simulink model "inventerthreephase"  (Simulink 7.3)
settings: Solver=ode45  StartTime=0.0  StopTime=0.2  RelTol=1e-3
libraries: powerlib x16
settings Model: Creator=Administrator  LastModifiedBy=Administrator

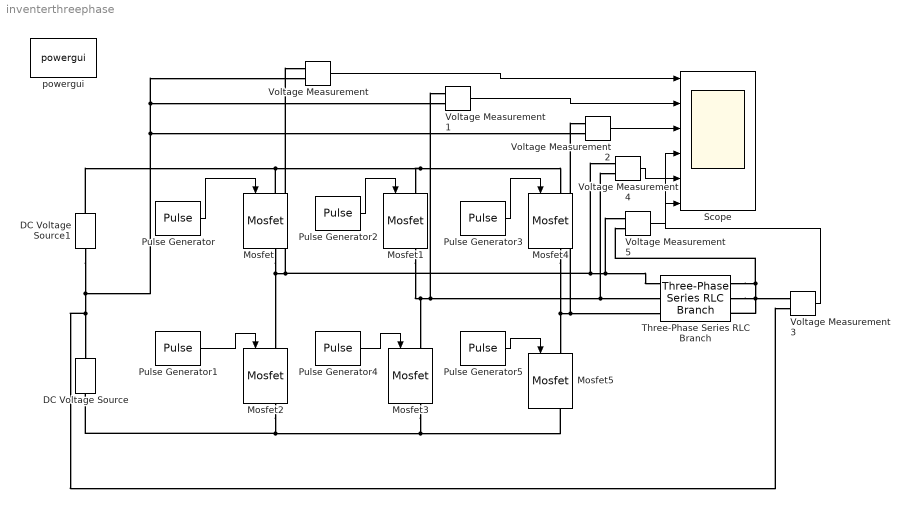
== system inventerthreephase ==
  DC Voltage Source : powerlib/Electrical Sources/DC Voltage Source  DialogController=POWERSYS.PowerSysDialog  SystemSampleTime=-1  Amplitude=100  Measurements=None
  DC Voltage Source1 : powerlib/Electrical Sources/DC Voltage Source  DialogController=POWERSYS.PowerSysDialog  SystemSampleTime=-1  Amplitude=100  Measurements=None
  Mosfet{,1..5} (6 alike) : powerlib/Power Electronics/Mosfet  DialogController=POWERSYS.PowerSysDialog  SystemSampleTime=-1  Ron=0.1  Lon=0  Rd=0.01  Vfd=0  IC=0  Rs=1e5  Cs=inf  Measurements=on
  Pulse Generator : DiscretePulseGenerator  PulseType=Time based  Amplitude=1  Period=0.02  PulseWidth=50  PhaseDelay=0  SampleTime=1
  Pulse Generator1 : DiscretePulseGenerator  PulseType=Time based  Amplitude=1  Period=0.02  PulseWidth=50  PhaseDelay=0.01  SampleTime=1
  Pulse Generator2 : DiscretePulseGenerator  PulseType=Time based  Amplitude=1  Period=0.02  PulseWidth=50  PhaseDelay=1/3*0.02  SampleTime=1
  Pulse Generator3 : DiscretePulseGenerator  PulseType=Time based  Amplitude=1  Period=0.02  PulseWidth=50  PhaseDelay=2/3*0.02  SampleTime=1
  Pulse Generator4 : DiscretePulseGenerator  PulseType=Time based  Amplitude=1  Period=0.02  PulseWidth=50  PhaseDelay=0.01+1/3*0.02  SampleTime=1
  Pulse Generator5 : DiscretePulseGenerator  PulseType=Time based  Amplitude=1  Period=0.02  PulseWidth=50  PhaseDelay=0.01+2/3*0.02  SampleTime=1
  Scope : Scope  NumInputPorts=6
      settings: YMin=-5~-5~-5~-5~-5~-5  YMax=5~5~5~5~5~5
  Three-Phase Series RLC Branch : powerlib/Elements/Three-Phase Series RLC Branch  DialogController=POWERSYS.PowerSysDialog  PhysicalDomain=powersysdomain  SubClassName=unknown  LeftPortType=p1  RightPortType=p1  LConnTagsString=A|B|C  RConnTagsString=A|B|C  BranchType=RL  Resistance=10  Inductance=0.01  Capacitance=1e-6  Measurements=None
  Voltage Measurement{,1..5} (6 alike) : powerlib/Measurements/Voltage Measurement  DialogController=POWERSYS.PowerSysDialog  SystemSampleTime=-1  PhasorSimulation=off  OutputType=Complex  PSBequivalent=0
  powergui : powerlib/powergui  Priority=1  SystemSampleTime=-1  SimulationMode=Continuous  SampleTime=50e-6  frequency=60  SPID=off  DisableSnubberDevices=off  DisableRonSwitches=off  DisableVfSwitches=off  SwTol=0  Interpol=off  frequencyindice=0  echomessages=off  HookPort=off  DisplayEquations=off  FunctionMessages=off  EnableUseOfTLC=off  x0status=blocks  RestoreLinks=warning  Frange=[0:2:500]  Ylog=off  Xlog=on  ShowGrid=off  save=off  variable=ZData  ZoomFFT=on  StartTime=0.0  cycles=1  DisplayStyle=1  fundamental=60  FreqAxis=off  MaxFrequency=1000  frequencyindicesteady=1  RmsSteady=1  display=off  Ts=0  methode=off
  wires:
  Pulse Generator/1 -> Mosfet/1
  Pulse Generator1/1 -> Mosfet2/1
  Pulse Generator2/1 -> Mosfet1/1
  Pulse Generator3/1 -> Mosfet4/1
  Pulse Generator4/1 -> Mosfet3/1
  Pulse Generator5/1 -> Mosfet5/1
  Voltage Measurement/1 -> Scope/1
  Voltage Measurement1/1 -> Scope/2
  Voltage Measurement2/1 -> Scope/3
  Voltage Measurement3/1 -> Scope/4
  Voltage Measurement4/1 -> Scope/5
  Voltage Measurement5/1 -> Scope/6
  connections:
  DC Voltage Source1/LConn1 -- Voltage Measurement/LConn2 -- Voltage Measurement1/LConn2 -- Voltage Measurement2/LConn2 -- DC Voltage Source/RConn1 -- Voltage Measurement3/LConn2
  Mosfet/RConn1 -- Mosfet2/LConn1 -- Voltage Measurement/LConn1 -- Voltage Measurement4/LConn1 -- Three-Phase Series RLC Branch/LConn1 -- Voltage Measurement5/LConn1
  Mosfet1/RConn1 -- Mosfet3/LConn1 -- Three-Phase Series RLC Branch/LConn2 -- Voltage Measurement4/LConn2 -- Voltage Measurement1/LConn1
  Mosfet4/RConn1 -- Mosfet5/LConn1 -- Three-Phase Series RLC Branch/LConn3 -- Voltage Measurement2/LConn1
  Mosfet/LConn1 -- Mosfet4/LConn1 -- Mosfet1/LConn1 -- DC Voltage Source1/RConn1
  Mosfet2/RConn1 -- Mosfet5/RConn1 -- Mosfet3/RConn1 -- DC Voltage Source/LConn1
  Three-Phase Series RLC Branch/RConn1 -- Three-Phase Series RLC Branch/RConn3 -- Three-Phase Series RLC Branch/RConn2 -- Voltage Measurement3/LConn1 -- Voltage Measurement5/LConn2
